simulink model "simulink_estanques"  (R2021a)
settings: Solver=ode1  StartTime=0.0  StopTime=10.0  FixedStep=0.001  RelTol=1e-3
settings Model: Creator=danie  LastModifiedBy=zeta

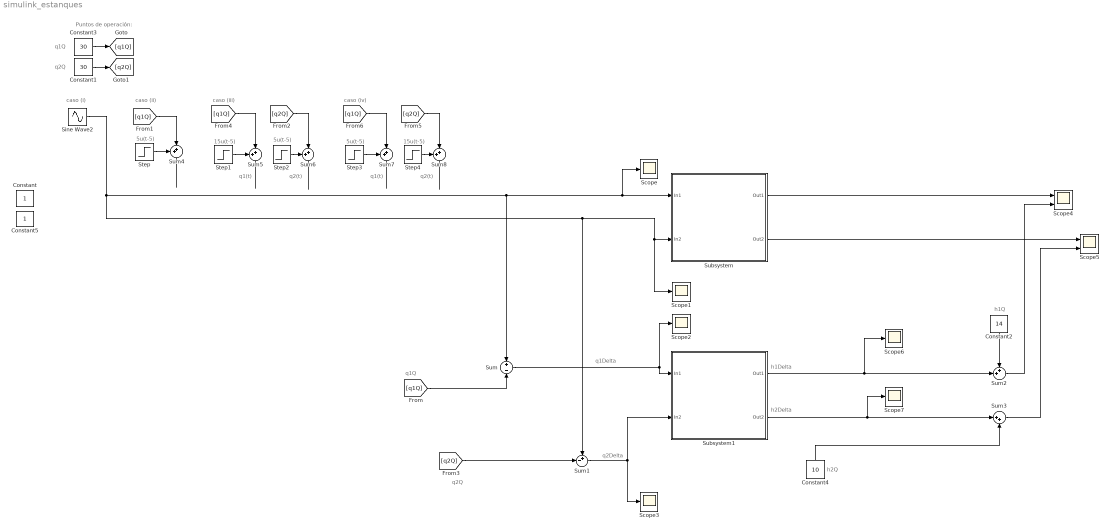
== system simulink_estanques ==
  note: 5u(t-5)
  note: 15u(t-5)
  note: q2(t)
  note: q1(t)
  note: caso (iii)
  note: caso (i)
  note: q2Q
  note: q1Q
  note: Puntos de operación:
  note: caso (ii)
  note: h2Delta
  note: h1Delta
  note: h1Q
  note: q1Delta
  note: q2Delta
  note: q2Q
  note: q1Q
  note: h2Q
  note: caso (iv)
  note: q1(t)
  note: q2(t)
  note: 15u(t-5)
  note: 5u(t-5)
  note: 5u(t-5)
  Constant : Constant
  Constant1 : Constant  Value=30
  Constant2 : Constant  Value=14
  Constant3 : Constant  Value=30
  Constant4 : Constant  Value=10
  Constant5 : Constant
  Scope{,1..3,6..7} (6 alike) : Scope
  Scope4 : Scope  NumInputPorts=2
  Scope5 : Scope  NumInputPorts=2
  Sine Wave2 : Sin  Amplitude=15  Bias=30  SampleTime=0
  Step : Step  Time=5  After=5  SampleTime=0
  Step1 : Step  Time=5  After=15  SampleTime=0
  Step2 : Step  Time=5  After=5  SampleTime=0
  Step3 : Step  Time=5  After=5  SampleTime=0
  Step4 : Step  Time=5  After=15  SampleTime=0
  Subsystem : Subsystem  mask{K=15, A=100, h10=14, h20=10}
      mask prompts: K "Coeficente de Traspaso"; A "Área Basal"; h10 "Altura inicial 1"; h20 "Altura inicial 2"
      mask Display:
      | port_label('input',1,'q1');
      | port_label('input',2,'q2');
      | port_label('output',1,'h1');
      | port_label('output',2,'h2');
      | fprintf('Sistema No lineal');
  Subsystem1 : Subsystem  mask{h2q=10, h1q=14, gamma=15/(2*(14-10)), K=15, A=100}
      mask prompts: K "Ka"; A "Área Basal"
      mask Display:
      | port_label('input',1,'q1');
      | port_label('input',2,'q2');
      | port_label('output',1,'h1');
      | port_label('output',2,'h2');
      | fprintf('Sistema Lineal');
  Sum : Sum  Inputs=+|-
  Sum1 : Sum  Inputs=+-|
  Sum{2,4..8} (6 alike) : Sum  Inputs=++|
  Sum3 : Sum  Inputs=|++
  wires:
  Sine Wave2/1 -> Scope1/1, Subsystem/2(In2), Sum1/1, Sum/1, Scope/1, Subsystem/1(In1)
  Sum/1 -> Scope2/1, Subsystem1/1(In1)
  [q2Q] -> Sum1/2
  Sum1/1 -> Subsystem1/2(In2), Scope3/1
  Subsystem1/2(Out2) -> Sum3/1, Scope7/1
  Subsystem1/1(Out1) -> Scope6/1, Sum2/2
  Constant4/1 -> Sum3/2
  Constant2/1 -> Sum2/1
  Sum2/1 -> Scope4/2
  Subsystem/1(Out1) -> Scope4/1
  Subsystem/2(Out2) -> Scope5/1
  Sum3/1 -> Scope5/2
  Step/1 -> Sum4/1
  Constant3/1 -> [q1Q]
  [q1Q] -> Sum4/2
  [q1Q] -> Sum/2
  Sum4/1 -> ?
  Constant1/1 -> [q2Q]
  Step1/1 -> Sum5/1
  [q1Q] -> Sum5/2
  Sum5/1 -> ?
  Step2/1 -> Sum6/1
  [q2Q] -> Sum6/2
  Sum6/1 -> ?
  Step4/1 -> Sum8/1
  [q1Q] -> Sum7/2
  Sum7/1 -> ?
  Sum8/1 -> ?
  [q2Q] -> Sum8/2
  Step3/1 -> Sum7/1

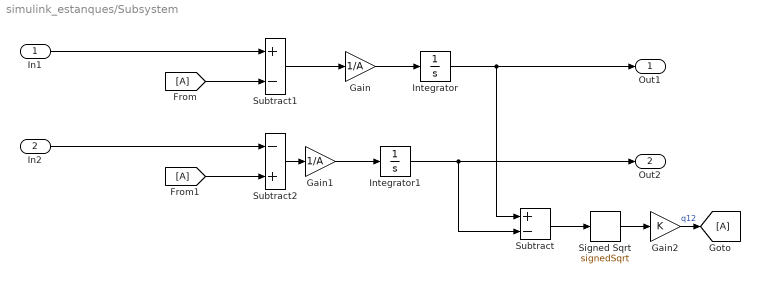
== system simulink_estanques/Subsystem ==
  In1 : Inport
  In2 : Inport  Port=2
  Gain : Gain  Gain=1/A
  Gain1 : Gain  Gain=1/A
  Gain2 : Gain  Gain=K
  Integrator : Integrator  InitialCondition=h10
  Integrator1 : Integrator  InitialCondition=h20
  Signed Sqrt : Sqrt  Operator=signedSqrt  SaturateOnIntegerOverflow=on
  Subtract : Sum  Inputs=+-
  Subtract1 : Sum  Inputs=+-
  Subtract2 : Sum  Inputs=-+
  Out1 : Outport
  Out2 : Outport  Port=2
  wires:
  Subtract/1 -> Signed Sqrt/1
  Signed Sqrt/1 -> Gain2/1
  In1/1 -> Subtract1/1
  Gain2/1 -> [A]  "q12"
  [A] -> Subtract1/2
  [A] -> Subtract2/2
  In2/1 -> Subtract2/1
  Integrator/1 -> Subtract/1, Out1/1
  Subtract1/1 -> Gain/1
  Gain/1 -> Integrator/1
  Subtract2/1 -> Gain1/1
  Gain1/1 -> Integrator1/1
  Integrator1/1 -> Out2/1, Subtract/2

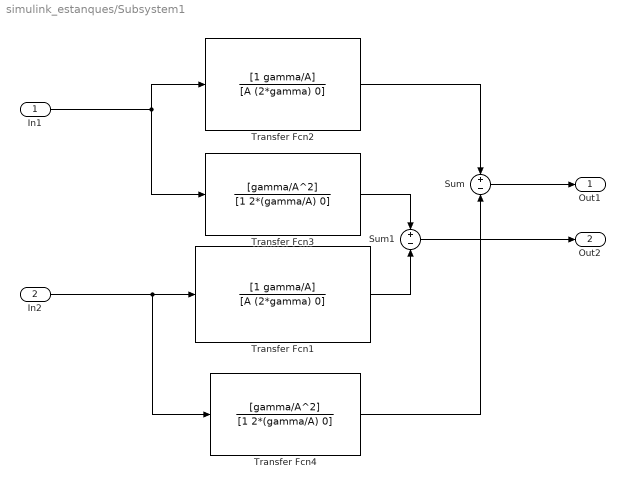
== system simulink_estanques/Subsystem1 ==
  In1 : Inport
  In2 : Inport  Port=2
  Sum : Sum  Inputs=+|-
  Sum1 : Sum  Inputs=+|-
  Transfer Fcn1 : TransferFcn  Numerator=[1 gamma/A]  Denominator=[A (2*gamma) 0]
  Transfer Fcn2 : TransferFcn  Numerator=[1 gamma/A]  Denominator=[A (2*gamma) 0]
  Transfer Fcn3 : TransferFcn  Numerator=[gamma/A^2]  Denominator=[1 2*(gamma/A) 0]
  Transfer Fcn4 : TransferFcn  Numerator=[gamma/A^2]  Denominator=[1 2*(gamma/A) 0]
  Out1 : Outport
  Out2 : Outport  Port=2
  wires:
  In1/1 -> Transfer Fcn3/1, Transfer Fcn2/1
  Transfer Fcn2/1 -> Sum/1
  Transfer Fcn3/1 -> Sum1/1
  Sum/1 -> Out1/1
  Sum1/1 -> Out2/1
  In2/1 -> Transfer Fcn4/1, Transfer Fcn1/1
  Transfer Fcn1/1 -> Sum1/2
  Transfer Fcn4/1 -> Sum/2
